simulink model "SimulationNumericalDif"  (Simulink 9.2)
settings: Solver=ode1  StartTime=0.0  StopTime=15  FixedStep=T  RelTol=1e-3  EnableMultiTasking=on
values from neighbouring files (symbols this model uses):
  K = place(A,B,p)    [StateFeedback_Controller_Observer_Design.m]    (also in equilibriumpositon_2_realsim.mat = [3103.64468197 1789.25362632 433.04949119 3.48374472995])
  Parameters = [11.9253 0.4203 0.1455 7.2462 1.8150 35.1492 0.0089]    [StateFeedback_Controller_Observer_Design.m]    (also in equilibriumpositon_2_realsim.mat = [11.9253 0.4203 0.1455 7.2462 1.815 35.1492 0.0089])
  q1 = x(1)    [NonLinModel.m]    (also in StateFeedback_Controller_Observer_Design.m = 1.57079632679; equilibriumpositon_2_realsim.mat = 1.57079632679)
  q2 = x(2)    [NonLinModel.m]    (also in StateFeedback_Controller_Observer_Design.m = 0; equilibriumpositon_2_realsim.mat = 3.14159265359)
  X0 = [q1+.1 q2-.2 0 0]    [StateFeedback_Controller_Observer_Design.m]    (also in equilibriumpositon_2_realsim.mat = [1.67079632679 2.94159265359 0 0])
settings Model: Creator=jafarm2  LastModifiedBy=AndyA  ExtModeTrigDuration=5000
settings SolverCC: PositivePriorityOrder=on
settings OptimizationCC: ExpressionDepthLimit=2147483647
settings DebuggingCC: SolverPrmCheckMsg=warning
settings RTWCC: SystemTargetFile=quarc_win64.tlc  TemplateMakefile=quarc_default_tmf  Description=QUARC Win64 Target
settings STFCustomTargetCC: TargetPreCompLibLocation=C:\PROGRA~3\QUARC\lib\2011b\win64\release  GeneratePreprocessorConditionals=Disable all  CPPClassGenCompliant=on  SystemTargetFile=quarc_win64.tlc
settings GRTTargetCC: TargetPreCompLibLocation=C:\PROGRA~3\QUARC\lib\2011b\win64\release  ParMdlRefBuildCompliant=off  CompOptLevelCompliant=off  ConcurrentExecutionCompliant=off  MatFileLogging=off  UseToolchainInfoCompliant=off  ExtMode=on  ExtModeMexFile=quarc_comm

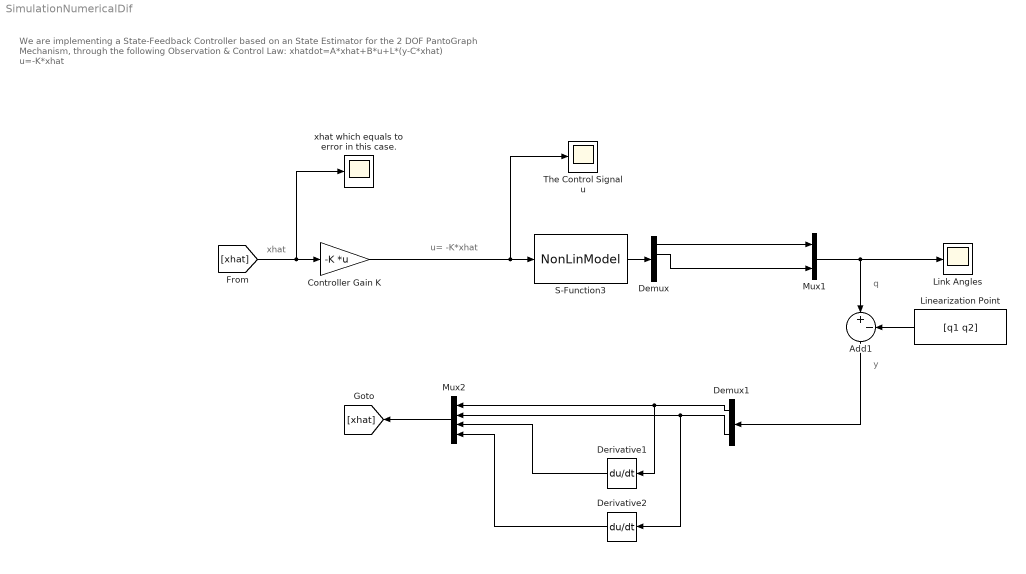
== system SimulationNumericalDif ==
  note: q
  note: y
  note: u= -K*xhat
  note: xhat
  note: We are implementing a State-Feedback Controller based on an State Estimator for the 2 DOF PantoGraph Mechanism,
      | through the following Observation & Control Law:
      | xhatdot=A*xhat+B*u+L*(y-C*xhat)
      | u=-K*xhat
  Add1 : Sum  Inputs=|+-
  Controller Gain K : Gain  Gain=-K  Multiplication=Matrix(K*u)
  Demux : Demux
  Demux1 : Demux  Outputs=2
  Derivative1 : Derivative
  Derivative2 : Derivative
  Linearization Point : Constant  Value=[q1 q2]
  Link Angles : Scope
  Mux1 : Mux  Inputs=2
  Mux2 : Mux
  S-Function3 : S-Function  FunctionName=NonLinModel  Parameters=X0,Parameters  SFunctionDeploymentMode=off  EnableBusSupport=off
  The Control Signal u : Scope
  xhat which equals to error in this case. : Scope
  wires:
  Controller Gain K/1 -> The Control Signal u/1, S-Function3/1
  Mux1/1 -> Link Angles/1, Add1/1
  Demux/1 -> Mux1/1
  Demux/2 -> Mux1/2
  Linearization Point/1 -> Add1/2
  [xhat] -> Controller Gain K/1, xhat which equals to error in this case./1
  S-Function3/1 -> Demux/1
  Add1/1 -> Demux1/1
  Demux1/1 -> Derivative1/1, Mux2/1
  Demux1/2 -> Derivative2/1, Mux2/2
  Derivative1/1 -> Mux2/3
  Derivative2/1 -> Mux2/4
  Mux2/1 -> [xhat]
